simulink model "Modelo_Simulacao2"  (Simulink 7.5)
settings: Solver=ode4  StartTime=0.0  StopTime=10  FixedStep=.005  RelTol=1e-3
settings Model: Creator=Leonardo  LastModifiedBy=Leo
settings OptimizationCC: InlineInvariantSignals=on  InitFltsAndDblsToZero=on
settings DebuggingCC: SaveWithParameterizedLinksMsg=none  SignalResolutionControl=TryResolveAllWithWarning  MultiTaskDSMMsg=warning  MultiTaskCondExecSysMsg=none  StrictBusMsg=None
settings RTWCC: IncludeERTFirstTime=on
settings GRTTargetCC: TargetFcnLib=ansi_tfl_tmw.mat

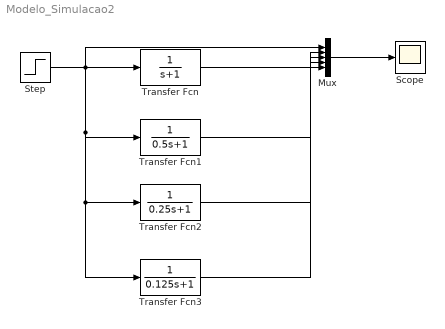
== system Modelo_Simulacao2 ==
  Mux : Mux  Inputs=5
  Scope : Scope
  Step : Step  Time=0  SampleTime=0
  Transfer Fcn : TransferFcn  Denominator=[1 1]
  Transfer Fcn1 : TransferFcn  Denominator=[0.5 1]
  Transfer Fcn2 : TransferFcn  Denominator=[0.25 1]
  Transfer Fcn3 : TransferFcn  Denominator=[0.125 1]
  wires:
  Step/1 -> Transfer Fcn/1, Mux/1, Transfer Fcn1/1, Transfer Fcn2/1, Transfer Fcn3/1
  Mux/1 -> Scope/1
  Transfer Fcn/1 -> Mux/2
  Transfer Fcn1/1 -> Mux/3
  Transfer Fcn2/1 -> Mux/4
  Transfer Fcn3/1 -> Mux/5
